simulink model "Ver001"  (R2016a)
settings: Solver=FixedStepAuto  StartTime=0.0  StopTime=inf  FixedStep=0.001  RelTol=1e-3
undefined symbols (not defined in the file): serial, Serial_Port, Standard_Devices
libraries: sldrtlib x5, instrumentlib x5, hdlsllib x2
settings Model: xpc_rtwmakecfg_data=_xpcnblib_  Creator=gadis  LastModifiedBy=gadis

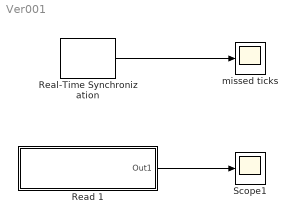
== system Ver001 ==
  Read 1 : Subsystem
  Real-Time Synchronization : sldrtlib/Real-Time Synchronization  SampleTime=1  MaxMissedTicks=10  ShowMissedTicks=on  YieldWhenWaiting=off
  Scope1 : Scope
  missed ticks : Scope
  wires:
  Real-Time Synchronization/1 -> missed ticks/1
  Read 1/1(Out1) -> Scope1/1

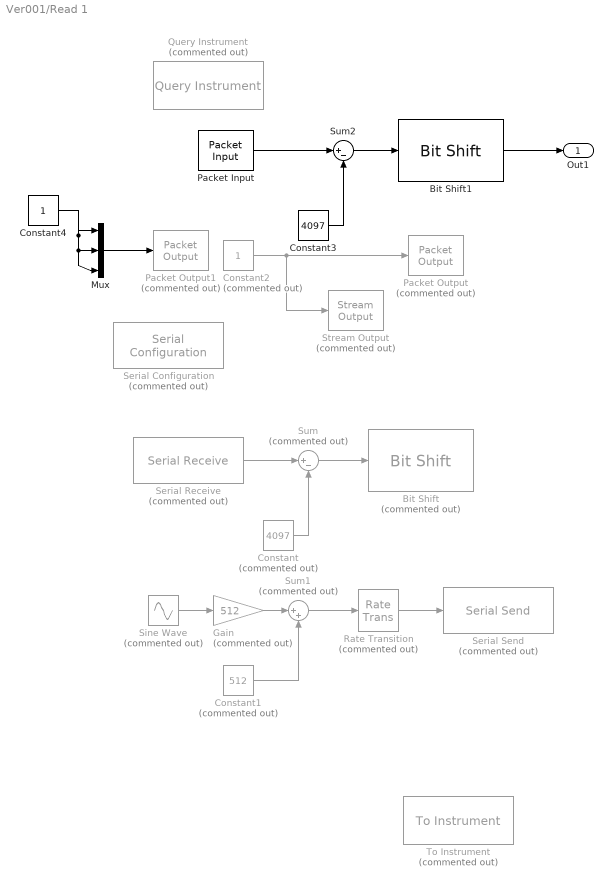
== system Ver001/Read 1 ==
  Bit Shift : hdlsllib/HDL Operations/Bit Shift  Commented=on  mode=Shift Right Arithmetic  N=1
  Bit Shift1 : hdlsllib/HDL Operations/Bit Shift  mode=Shift Right Arithmetic  N=1
  Constant : Constant  Commented=on  Value=4097
  Constant1 : Constant  Commented=on  Value=512
  Constant2 : Constant  Commented=on
  Constant3 : Constant  Value=4097
  Constant4 : Constant
  Gain : Gain  Commented=on  Gain=512
  Mux : Mux  Inputs=3
  Packet Input : sldrtlib/Packet Input  SampleTime=0.01  MaxMissedTicks=10  ShowMissedTicks=off  YieldWhenWaiting=off  DrvName=Standard_Devices/Serial_Port  DrvAddress=3  DrvOptions=[256000 8 0 0 0 0 0 0]  PacketSize=4  DataTypes='2*uint16'  ShowReady=off  ShowError=off  PacketID=1  ByteOrder=1  ShowTimestamp=off
      settings: AttributesFormatString=Standard Devices\nSerial Port [3h]
  Packet Output : sldrtlib/Packet Output  Commented=on  SampleTime=0.02  MaxMissedTicks=10  ShowMissedTicks=off  YieldWhenWaiting=off  DrvName=Standard_Devices/Serial_Port  DrvAddress=3  DrvOptions=[256000 8 0 0 0 0 0 0]  PacketSize=1  DataTypes='uint8'  ShowReady=off  ShowError=off  PacketID=1  ByteOrder=1  InitialValue=[]  FinalValue=[]
      settings: AttributesFormatString=Standard Devices\nSerial Port [3h]
  Packet Output1 : sldrtlib/Packet Output  Commented=on  SampleTime=0.1  MaxMissedTicks=10  ShowMissedTicks=off  YieldWhenWaiting=off  DrvName=Standard_Devices/Serial_Port  DrvAddress=5  DrvOptions=[9600 8 0 0 0 0 0 0]  PacketSize=3  DataTypes='3*uint8'  ShowReady=off  ShowError=off  PacketID=1  ByteOrder=1  InitialValue=[1 1 1]  FinalValue=[]
      settings: AttributesFormatString=Standard Devices\nSerial Port [5h]
  Query Instrument : instrumentlib/Query Instrument  Commented=on  sampleTime=0.005  isWorkspaceObject=off  timeout=10  inputBufferSize=512  protocol=Serial  serialPort=COM3  baudRate=115200  gpibVendor=Agilent Technologies  boardIndex=0  primaryAddress=1  secondaryAddress=0  visaVendor=Agilent  visaSerialPort=0  chassisIndex=0  logicalAddress=0  tcpRemoteHost='127.0.0.1'  tcpRemotePort=4500  udpRemoteHost='127.0.0.1'  udpRemotePort=9090  visaTCPBoardIndex=0  visaTCPRemoteHost='127.0.0.1'  usbBoardIndex=0  usbManufID=0  usbModelCode=0  usbSerialNumber=0  initAction=None  initCommand='DATA:SOURCE CH1'  initFunction=get  queryCommand='1'  responseFormat=Binary  asciiFormatting='%d,'  precision=16-bit unsigned integer  byteOrder=Little Endian  valuesToRead=1  removeBytes=off  afterOutputAction=Repeat query for new data  enableFrames=on  frameSize=2
  Rate Transition : RateTransition  Commented=on
  Serial Configuration : instrumentlib/Serial Configuration  Priority=-200000  Commented=on  ComPortMenu=<Please select a port...>  ComPort=COM3  ObjConstructor=serial('COM3');  BaudRate=115200  DataBits=8  Parity=none  StopBits=1  FlowControl=none  Timeout=10  ByteOrder=LittleEndian
  Serial Receive : instrumentlib/Serial Receive  Commented=on  ComPortMenu=<Please select a port...>  ComPort=COM3  ObjConstructor=serial('COM3');  Terminator=<none>  DataSize="[2  2]"  DataType=uint16  EnableBlockingMode=on  ActionDataUnavailable=Output last received value  CustomValue=0  SampleTime=0.1
  Serial Send : instrumentlib/Serial Send  Commented=on  ComPortMenu=<Please select a port...>  ComPort=COM3  ObjConstructor=serial('COM3');  Header=1  Terminator=<none>  EnableBlockingMode=on
  Sine Wave : Sin  Commented=on  SampleTime=0
  Stream Output : sldrtlib/Stream Output  Commented=on  SampleTime=0.02  MaxMissedTicks=10  ShowMissedTicks=off  YieldWhenWaiting=off  DrvName=Standard_Devices/Serial_Port  DrvAddress=3  DrvOptions=[256000 8 0 0 0 0 0 0]  PortSizes=1  FormatString='%x'  ShowReady=off  ShowError=off  InitialValue=[]  FinalValue=[]
      settings: AttributesFormatString=Standard Devices\nSerial Port [3h]
  Sum : Sum  Commented=on  Inputs=|+-
  Sum1 : Sum  Commented=on  Inputs=|++
  Sum2 : Sum  Inputs=|+-
  To Instrument : instrumentlib/To Instrument  Commented=on  sampleTime=-1  isWorkspaceObject=off  timeout=10  inputBufferSize=8192  protocol=Serial  serialPort=COM3  baudRate=115200  gpibVendor=Agilent Technologies  boardIndex=0  primaryAddress=1  secondaryAddress=0  visaVendor=Agilent  visaSerialPort=0  chassisIndex=0  logicalAddress=0  tcpRemoteHost='127.0.0.1'  tcpRemotePort=4500  udpRemoteHost='127.0.0.1'  udpRemotePort=9090  visaTCPBoardIndex=0  visaTCPRemoteHost='127.0.0.1'  usbBoardIndex=0  usbManufID=0  usbModelCode=0  usbSerialNumber=0  initAction=None  initCommand='DATA:SOURCE CH1'  initFunction=get  command=''  sendFormat=Binary  asciiFormatting='%d'  precision=8-bit integer  byteOrder=Little Endian
  Out1 : Outport
  wires:
  Constant/1 -> Sum/2
  Sum/1 -> Bit Shift/1
  Serial Receive/1 -> Sum/1
  Sine Wave/1 -> Gain/1
  Gain/1 -> Sum1/1
  Constant1/1 -> Sum1/2
  Sum1/1 -> Rate Transition/1
  Rate Transition/1 -> Serial Send/1
  Constant2/1 -> Stream Output/1, Packet Output/1
  Constant3/1 -> Sum2/2
  Sum2/1 -> Bit Shift1/1
  Constant4/1 -> Mux/3, Mux/2, Mux/1
  Mux/1 -> Packet Output1/1
  Bit Shift1/1 -> Out1/1
  Packet Input/1 -> Sum2/1
